simulink model "mconversion1"  (Simulink 6.0)
settings: Solver=ode3  StartTime=0.0  StopTime=10.0  FixedStep=0.7  RelTol=1e-3
libraries: lib5 x1, lib2 x1, lib4 x1, lib3 x1, lib1 x1
settings Model: Creator=awarlock  LastModifiedBy=awarlock  ExtModeAutoUpdateStatusClock=off
settings DataIOCC: SignalLoggingName=logsOut
settings OptimizationCC: InlineParams=on
settings DebuggingCC: CheckExecutionContextPreStartOutputMsg=on  CheckExecutionContextRuntimeOutputMsg=on  SolverPrmCheckMsg=none
settings HardwareCC: TargetUnknown=on
settings RTWCC: SystemTargetFile=ert.tlc  TemplateMakefile=ert_default_tmf  ProcessScript=ert_make_rtw_hook
settings CodeAppCC: IgnoreCustomStorageClasses=off
settings ERTTargetCC: TargetFcnLib=ansi_tfl_tmw.mat  GenFloatMathFcnCalls=ANSI_C  GenerateSampleERTMain=on  LifeSpan=1  SupportContinuousTime=on  SupportNonInlinedSFcns=on  RootIOFormat=Individual Arguments  ERTCustomFileTemplate=example_file_process.tlc  InitialValueSource=Model
settings SFSimCC: SFSimApplyToAllLibs=on  SFSimBuildMode=Incremental

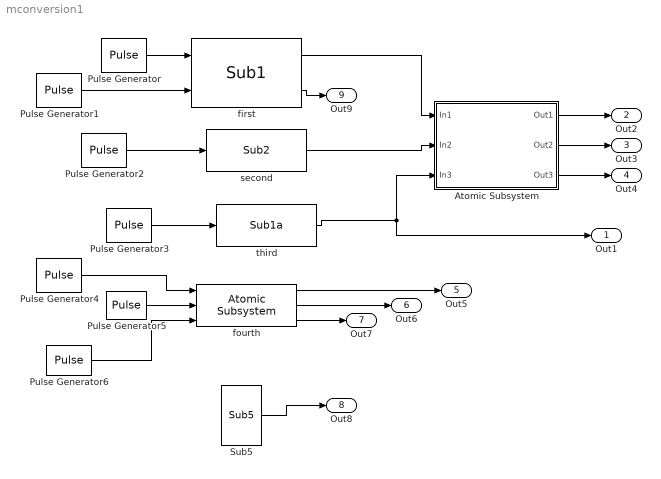
== system mconversion1 ==
  Atomic Subsystem : Subsystem  TreatAsAtomicUnit=on  PropExecContextAcrossSSBoundary=on
  Pulse Generator : DiscretePulseGenerator  SampleTime=0.7
  Pulse Generator1 : DiscretePulseGenerator  Period=3  SampleTime=0.7
  Pulse Generator2 : DiscretePulseGenerator  Period=3  PulseWidth=2  SampleTime=0.7
  Pulse Generator3 : DiscretePulseGenerator  Period=4  SampleTime=0.7
  Pulse Generator4 : DiscretePulseGenerator  Period=4  PulseWidth=2  SampleTime=0.7
  Pulse Generator5 : DiscretePulseGenerator  Period=4  PulseWidth=3  SampleTime=0.7
  Pulse Generator6 : DiscretePulseGenerator  Period=5  PulseWidth=3  SampleTime=0.7
  Sub5 : lib5/Sub5
  first : lib2/Sub1
  fourth : lib4/Atomic Subsystem
  second : lib3/Sub2
  third : lib1/Sub1a
  Out1 : Outport
  Out2 : Outport  Port=2
  Out3 : Outport  Port=3
  Out4 : Outport  Port=4
  Out5 : Outport  Port=5
  Out6 : Outport  Port=6
  Out7 : Outport  Port=7
  Out8 : Outport  Port=8
  Out9 : Outport  Port=9
  wires:
  Pulse Generator/1 -> first/1
  first/1 -> Atomic Subsystem/1(In1)
  second/1 -> Atomic Subsystem/2(In2)
  third/1 -> Atomic Subsystem/3(In3), Out1/1
  Atomic Subsystem/1(Out1) -> Out2/1
  Atomic Subsystem/2(Out2) -> Out3/1
  Atomic Subsystem/3(Out3) -> Out4/1
  Pulse Generator1/1 -> first/2
  Pulse Generator2/1 -> second/1
  Pulse Generator3/1 -> third/1
  Pulse Generator4/1 -> fourth/1
  Pulse Generator5/1 -> fourth/2
  Pulse Generator6/1 -> fourth/3
  fourth/1 -> Out5/1
  fourth/2 -> Out6/1
  fourth/3 -> Out7/1
  Sub5/1 -> Out8/1
  first/2 -> Out9/1

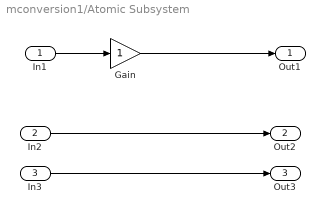
== system mconversion1/Atomic Subsystem ==
  In1 : Inport  LatchInput=off
  In2 : Inport  Port=2  LatchInput=off
  In3 : Inport  Port=3  LatchInput=off
  Gain : Gain
  Out1 : Outport
  Out2 : Outport  Port=2
  Out3 : Outport  Port=3
  wires:
  In1/1 -> Gain/1
  In2/1 -> Out2/1
  In3/1 -> Out3/1
  Gain/1 -> Out1/1
